simulink library "csu_gib_gdn_inertial_burn_lib"  (R2014b)
settings: Solver=ode45  StartTime=0.0  StopTime=10.0  RelTol=1e-3
undefined symbols (not defined in the file or in its folder): gdn_thruster_dur_min
settings Model: Creator=Nilesh  LastModifiedBy=mstewart

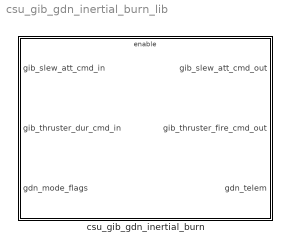
== system csu_gib_gdn_inertial_burn_lib ==
  csu_gib_gdn_inertial_burn : Subsystem

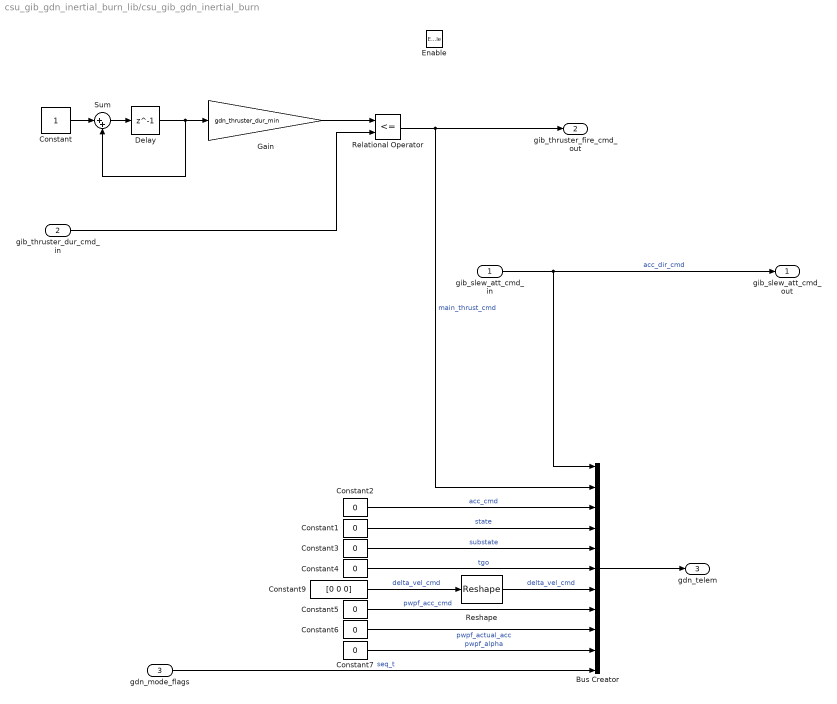
== system csu_gib_gdn_inertial_burn_lib/csu_gib_gdn_inertial_burn ==
  gib_slew_att_cmd_in : Inport
  gib_thruster_dur_cmd_in : Inport  Port=2
  gdn_mode_flags : Inport  Port=3
  Enable : EnablePort
  Bus Creator : BusCreator  Inputs=11  OutDataTypeStr=Bus: gdn_tlm_msg  NonVirtualBus=on
  Constant : Constant
  Constant{1..7} (7 alike) : Constant  Value=0
  Constant9 : Constant  Value=[0 0 0]
  Delay : Delay  DelayLength=1  InitialCondition=0
  Gain : Gain  Gain=gdn_thruster_dur_min
  Relational Operator : RelationalOperator  Operator=<=  OutDataTypeStr=boolean
  Reshape : Reshape  OutputDimensionality=Column vector (2-D)
  Sum : Sum  Inputs=|++
  gib_slew_att_cmd_out : Outport
  gib_thruster_fire_cmd_out : Outport  Port=2
  gdn_telem : Outport  Port=3
  wires:
  Constant/1 -> Sum/1
  gib_thruster_dur_cmd_in/1 -> Relational Operator/2
  Sum/1 -> Delay/1
  Delay/1 -> Sum/2, Gain/1
  Gain/1 -> Relational Operator/1
  Reshape/1 -> Bus Creator/7  "delta_vel_cmd"
  gdn_mode_flags/1 -> Bus Creator/11  "seq_t"
  Constant7/1 -> Bus Creator/10  "pwpf_alpha"
  Constant6/1 -> Bus Creator/9  "pwpf_actual_acc"
  Constant5/1 -> Bus Creator/8  "pwpf_acc_cmd"
  Constant9/1 -> Reshape/1  "delta_vel_cmd"
  Constant4/1 -> Bus Creator/6  "tgo"
  Constant3/1 -> Bus Creator/5  "substate"
  Constant1/1 -> Bus Creator/4  "state"
  Constant2/1 -> Bus Creator/3  "acc_cmd"
  gib_slew_att_cmd_in/1 -> Bus Creator/1, gib_slew_att_cmd_out/1  "acc_dir_cmd"
  Bus Creator/1 -> gdn_telem/1
  Relational Operator/1 -> Bus Creator/2, gib_thruster_fire_cmd_out/1  "main_thrust_cmd"
